simulink model "quadro_model_new_ast_time"  (R2020b)
settings: Solver=VariableStepAuto  StartTime=0.0  StopTime=20.0  RelTol=1e-3
values from neighbouring files (symbols this model uses):
  A1_1 = [0 1; 0 0]    [quadro_new_ast_test.m]
  A1_3 = [0 1 0 0; 0 0 9.8 0; 0 0 0 1; 0 0 0 0]    [quadro_new_ast_test.m]
  Bw = [B Bad]    [quadro_new_ast_test.m]
  C1_1 = [1 0]    [quadro_new_ast_test.m]
  C1_3 = [1 0 0 0; 0 0 1 0]    [quadro_new_ast_test.m]
  H1 = H1'    [quadro_new_ast_test.m]
  H3 = H3'    [quadro_new_ast_test.m]
  K4 = -K4    [quadro_new_ast_test.m]
  M1 = [w*mz*(A1_1-H1*C1_1) w*mz*B1_1 w*mz*H1+w*nz]    [quadro_new_ast_test.m]
  M3 = [w*mt*(A1_3-H3*C1_3) w*mt*B1_3 w*mt*H3+w*nt]    [quadro_new_ast_test.m]
  T1 = [B1_1 H1]    [quadro_new_ast_test.m]
  T3 = [B1_3 H3]    [quadro_new_ast_test.m]
  x0_0 = [0; 0; 0; 0; 0; 0; 0; 0; 0; 0; 0; 0]    [quadro_new_ast_test.m]
undefined symbols (not defined in the file or in its folder): A, B
settings Model: Creator=Наташа  LastModifiedBy=Наташа

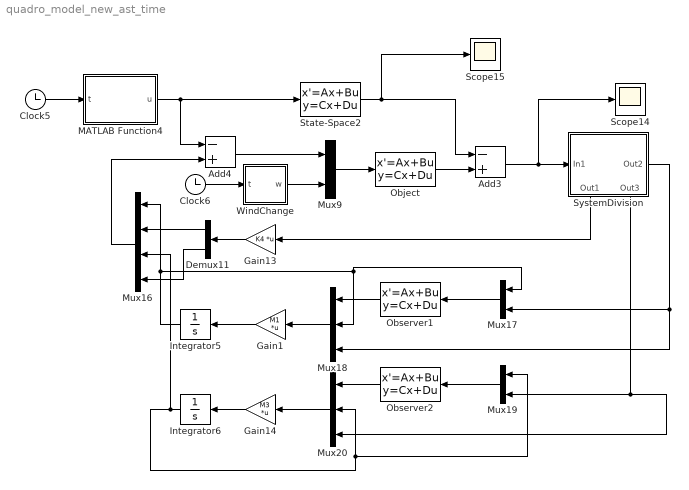
== system quadro_model_new_ast_time ==
  Add3 : Sum  Inputs=-+
  Add4 : Sum  Inputs=-+
  Clock5 : Clock
  Clock6 : Clock
  Demux11 : Demux  Outputs=2
  Gain1 : Gain  Gain=M1  Multiplication=Matrix(K*u) (u vector)
  Gain13 : Gain  Gain=K4  Multiplication=Matrix(K*u) (u vector)
  Gain14 : Gain  Gain=M3  Multiplication=Matrix(K*u) (u vector)
  Integrator5 : Integrator
  Integrator6 : Integrator
  MATLAB Function4 : MATLAB Function  TreatAsAtomicUnit=on
  Mux16 : Mux
  Mux17 : Mux  Inputs=2
  Mux18 : Mux  Inputs=3
  Mux19 : Mux  Inputs=2
  Mux20 : Mux  Inputs=3
  Mux9 : Mux  Inputs=2
  Object : StateSpace  A=A  B=Bw  C=eye(12)  D=zeros(12,6)  InitialCondition=x0_0
  Observer1 : StateSpace  A=A1_1-H1*C1_1  B=T1  C=eye(2)  D=zeros(2,2)  InitialCondition=0
  Observer2 : StateSpace  A=A1_3-H3*C1_3  B=T3  C=eye(4)  D=zeros(4,3)  InitialCondition=0
  Scope14 : Scope
  Scope15 : Scope
  State-Space2 : StateSpace  A=A  B=B  C=eye(12)  D=zeros(12,4)  InitialCondition=x0_0
  SystemDivision : Subsystem
      settings: PortSchema="{\"entries\":[{\"content\":{\"sides\":[{\"content\":{\"connectorIds\":[\"In1\"]},\"type\":\"ConnectorPlacement.EquallySpacedRectSide\",\"uuid\":\"9a4dcc1c-9aa9-4002-a8c7-2059fdadfec6\"},{\"content\":{\"connectorIds\":[\"Out1\"],\"side\":\"RIGHT\"},\"type\":\"ConnectorPlacement.EquallySpacedRectSide\",\"uuid\":\"2a70adff-7dff-4c4c-889c-0152b0f8b5f0\"},{\"content\":{\"connectorIds\":[],\"side\":\"TOP\"},\"type\":\"ConnectorPlacement.EquallySpacedRectSide\",\"uuid\":\"a8a436b6-dcb1-4d9b-a20e-4825be932de5\"},{\"content\":{\"connectorIds\":[\"Out2\",\"Out3\"],\"side\":\"BOTTOM\"},\"type\":\"ConnectorPlacement.EquallySpacedRectSide\",\"uuid\":\"cd26919a-5abd-48dc-8e9c-2050175e4448\"},{\"content\":{\"connectorIds\":[],\"side\":\"HIDDEN\"},\"type\":\"ConnectorPlacement.EquallySpacedRectSide\",\"uuid\":\"f1a9fd8c-b373-4d9e-8d44-62a8e17dbb8a\"}]},\"type\":\"ConnectorPlacement.EquallySpacedConnector\",\"uuid\":\"a01edf70-af93-4d9d-9478-f6e97764c621\"}],\"packageUris\":[\"http://schema.mathworks.com/mf0/Connector/R2020b\"],\"version\":\"1.0\"}"
  WindChange : MATLAB Function  TreatAsAtomicUnit=on
  wires:
  Gain1/1 -> Integrator5/1
  Integrator5/1 -> Mux16/1, Mux17/1, Mux18/2
  Gain14/1 -> Integrator6/1
  Integrator6/1 -> Mux19/1, Mux20/2, Mux16/3
  Mux20/1 -> Gain14/1
  Observer1/1 -> Mux18/1
  SystemDivision/1(Out2) -> Mux18/3, Mux17/2
  Mux9/1 -> Object/1
  Mux19/1 -> Observer2/1
  SystemDivision/3(Out3) -> Mux20/3, Mux19/2
  Add4/1 -> Mux9/1
  Demux11/1 -> Mux16/2
  Mux16/1 -> Add4/2
  WindChange/1(w) -> Mux9/2
  MATLAB Function4/1(u) -> Add4/1, State-Space2/1
  Clock5/1 -> MATLAB Function4/1(t)
  State-Space2/1 -> Add3/1, Scope15/1
  Demux11/2 -> Mux16/4
  Gain13/1 -> Demux11/1
  SystemDivision/2(Out1) -> Gain13/1
  Add3/1 -> Scope14/1, SystemDivision/1(In1)
  Clock6/1 -> WindChange/1(t)
  Object/1 -> Add3/2
  Observer2/1 -> Mux20/1
  Mux17/1 -> Observer1/1
  Mux18/1 -> Gain1/1

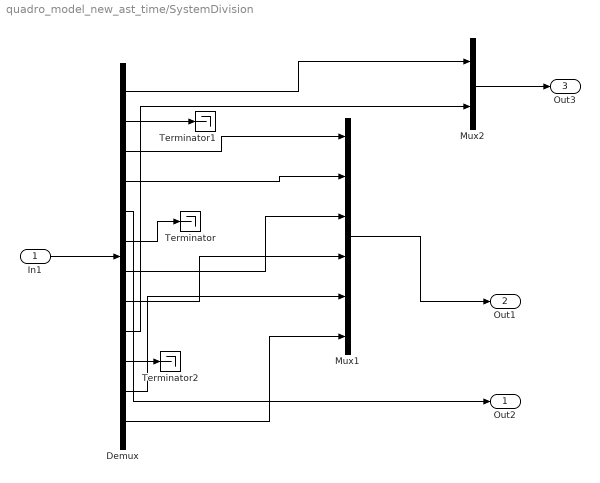
== system quadro_model_new_ast_time/SystemDivision ==
  In1 : Inport
  Demux : Demux  Outputs=12
  Mux1 : Mux  Inputs=6
  Mux2 : Mux  Inputs=2
  Terminator : Terminator
  Terminator1 : Terminator
  Terminator2 : Terminator
  Out2 : Outport
  Out1 : Outport  Port=2
  Out3 : Outport  Port=3
  wires:
  In1/1 -> Demux/1
  Mux1/1 -> Out1/1
  Demux/1 -> Mux2/1
  Demux/2 -> Terminator1/1
  Demux/3 -> Mux1/1
  Demux/4 -> Mux1/2
  Demux/7 -> Mux1/3
  Demux/8 -> Mux1/4
  Demux/9 -> Mux2/2
  Demux/10 -> Terminator2/1
  Demux/11 -> Mux1/5
  Demux/12 -> Mux1/6
  Demux/6 -> Terminator/1
  Demux/5 -> Out2/1
  Mux2/1 -> Out3/1

== matlab function quadro_model_new_ast_time/WindChange ==
  data: t input; w output
function w = fcn(t)

w = [1.5;10]*(t<=5) + [1;5]*(t>5&t<=10) + [1.2;7]*(t>10);

== matlab function quadro_model_new_ast_time/MATLAB Function4 ==
  data: t input; u output
function u = fcn(t)
u = zeros(4,1); 

% u(1,1) = 0.3 - 0.03*t;
% u(2,1) = 0; 
% u(3,1) = -9.8014e-6*t^3 + 0.00027017*t^2 - 0.001922*t + 0.0028004; 
% %u(4,1) = 0.00011781*t - 0.0011781; 
% u(4,1) = 0; 

% u(1,1) = 0.15 - 0.015*t;
% u(2,1) = 0; 
% u(3,1) = - 4.9007e-6*t^3 + 0.00013509*t^2 - 0.00096102*t + 0.0014002; 
% u(4,1) = 0; 

u(1,1) = 0.15 - 0.015*t;
u(2,1) = 0; 
u(3,1) = - 1.1634e-6*t^3 + 0.000033269*t^2 - 0.0002518*t + 0.00040888; 
u(4,1) = 0;
